simulink subsystem "GlobalMPController"  (R2022b)
settings: Solver=VariableStepAuto  StartTime=0.0  StopTime=10.0  RelTol=1e-3
model mask{c=0}
  mask prompts: c "standard constants"
settings Model: Creator=is123  LastModifiedBy=laula

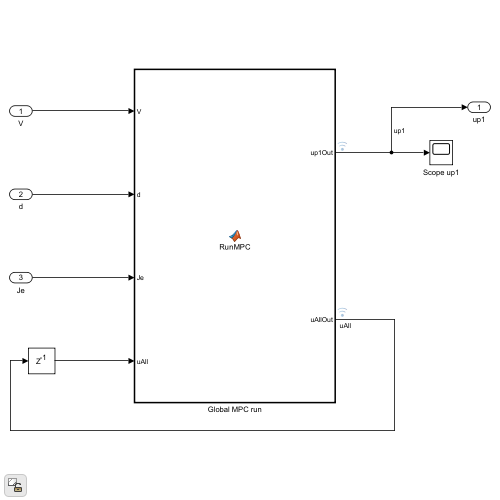
[thumbnail: Simulink's stored preview of the top-level diagram]
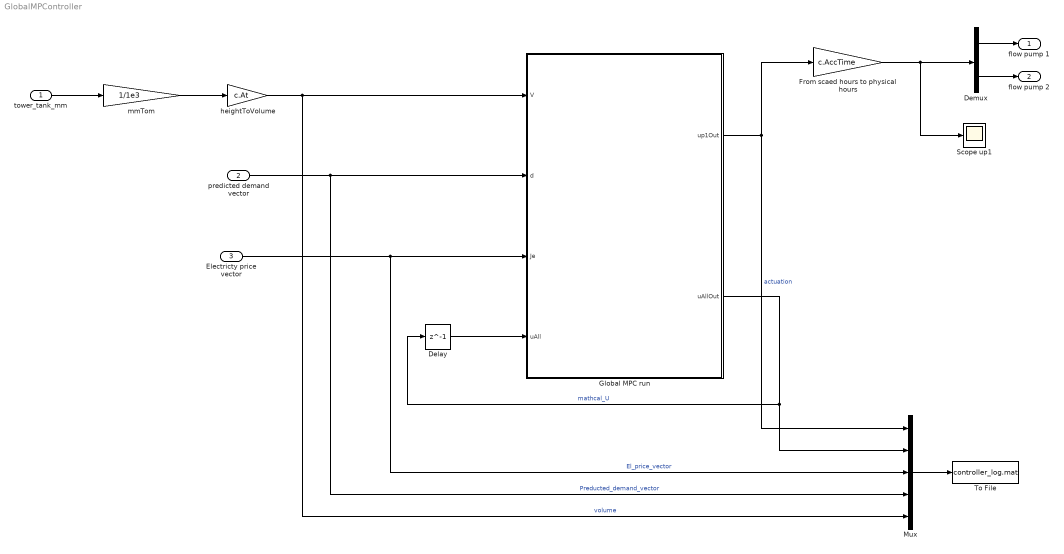
== system GlobalMPController ==
  tower_tank_mm : Inport
  predicted demand vector : Inport  Port=2
  Electricty price vector : Inport  Port=3
  Delay : Delay  DelayLength=1  InitialCondition=zeros(c.Nu*c.Nc,1)
  Demux : Demux  Outputs=2
  From scaed hours to physical hours : Gain  Gain=c.AccTime
  Global MPC run : MATLAB Function  TreatAsAtomicUnit=on  SystemSampleTime=3600/c.AccTime
  Mux : Mux  Inputs=5
  Scope up1 : Scope
  To File : ToFile  Filename=controller_log.mat  SaveFormat=Timeseries
  heightToVolume : Gain  Gain=c.At
  mmTom : Gain  Gain=1/1e3
  "flow pump 1 " : Outport
  flow pump 2 : Outport  Port=2
  wires:
  Global MPC run/1(up1Out) -> From scaed hours to physical hours/1, Mux/1  "actuation"
  Global MPC run/2(uAllOut) -> Delay/1, Mux/2  "mathcal_U"
  Delay/1 -> Global MPC run/4(uAll)
  predicted demand vector/1 -> Global MPC run/2(d), Mux/4  "Preducted_demand_vector"
  Electricty price vector/1 -> Global MPC run/3(Je), Mux/3  "El_price_vector"
  Demux/2 -> flow pump 2/1
  Demux/1 -> "flow pump 1 "/1
  heightToVolume/1 -> Global MPC run/1(V), Mux/5  "volume"
  tower_tank_mm/1 -> mmTom/1
  mmTom/1 -> heightToVolume/1
  From scaed hours to physical hours/1 -> Demux/1, Scope up1/1
  Mux/1 -> To File/1

== matlab function GlobalMPController/Global MPC run ==
  data: V input; d input; Je input; uAll input; up1Out output; uAllOut output
function [up1Out,uAllOut]= RunMPC(V,d, Je,uAll)
%needed to make the function run 
coder.extrinsic('mpcRun')
%Loading in standard Constants

%Need putting the demand, current water volume, and eletricity price into
%standard constants
data.V=V;
data.d=d;
data.Je=Je;

%Setting size of the output, neccesary to make Simulink run 
c=scaled_standard_constants;
up1Out=zeros(c.Nu,1);
uAllOut=zeros(c.Nu*c.Nc,1);



%solving the global model control problem 
[up1OutTemp,uAllOutTemp]=mpcRun(data,uAll); 
up1Out=up1OutTemp;
uAllOut=uAllOutTemp;
end
